simulink model "model_simulink"  (R2016b)
settings: Solver=FixedStepAuto  StartTime=0.0  StopTime=inf  MaxStep=8.0  RelTol=1e-3
undefined symbols (not defined in the file): Serial_Port, Standard_Devices
libraries: sldrtlib x1
settings Model: Creator=Vjekoslav  LastModifiedBy=Vjekoslav

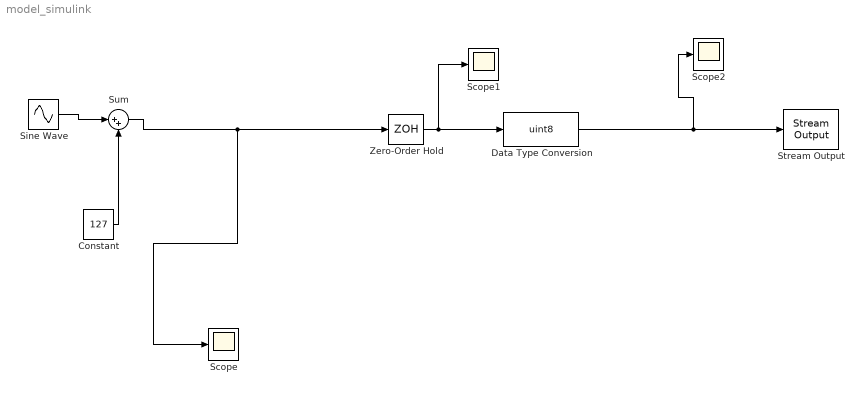
== system model_simulink ==
  Constant : Constant  Value=127
  Data Type Conversion : DataTypeConversion  OutMin=[0]  OutMax=[255]  OutDataTypeStr=uint8  RndMeth=Nearest
  Scope : Scope
  Scope1 : Scope
  Scope2 : Scope
  Sine Wave : Sin  Amplitude=127  Frequency=1/1  SampleTime=0
  Stream Output : sldrtlib/Stream Output  SampleTime=0.1  MaxMissedTicks=10  ShowMissedTicks=off  YieldWhenWaiting=off  DrvName=Standard_Devices/Serial_Port  DrvAddress=4  DrvOptions=[115200 8 0 0 0 0 0 0]  PortSizes=1  FormatString='%c'  ShowReady=off  ShowError=off  InitialValue=[]  FinalValue=[]
      settings: AttributesFormatString=Standard Devices\nSerial Port [4h]
  Sum : Sum  Inputs=|++
  Zero-Order Hold : ZeroOrderHold  SampleTime=-1
  wires:
  Sum/1 -> Scope/1, Zero-Order Hold/1
  Sine Wave/1 -> Sum/1
  Constant/1 -> Sum/2
  Zero-Order Hold/1 -> Data Type Conversion/1, Scope1/1
  Data Type Conversion/1 -> Stream Output/1, Scope2/1
